simulink model "ijc_template"  (R2020a)
settings: Solver=ode4  StartTime=0.0  StopTime=100  FixedStep=dt  RelTol=1e-3
undefined symbols (not defined in the file): g, Gv, Jm, K, kd1, kd2, ki, kp, Kt, Kv, l1, lc1, lc2, m1, m2, Ra
libraries: simulink x8
settings Model: Creator=baradaran  LastModifiedBy=User
settings DataIOCC: ReturnWorkspaceOutputs=off
settings DebuggingCC: ArithmeticOperatorsInVariantConditions=warning
settings SFSimCC: SimUseLocalCustomCode=off  CustomCodeUndefinedFunction=UseInterfaceOnly
settings RTWCC: RTWUseLocalCustomCode=off

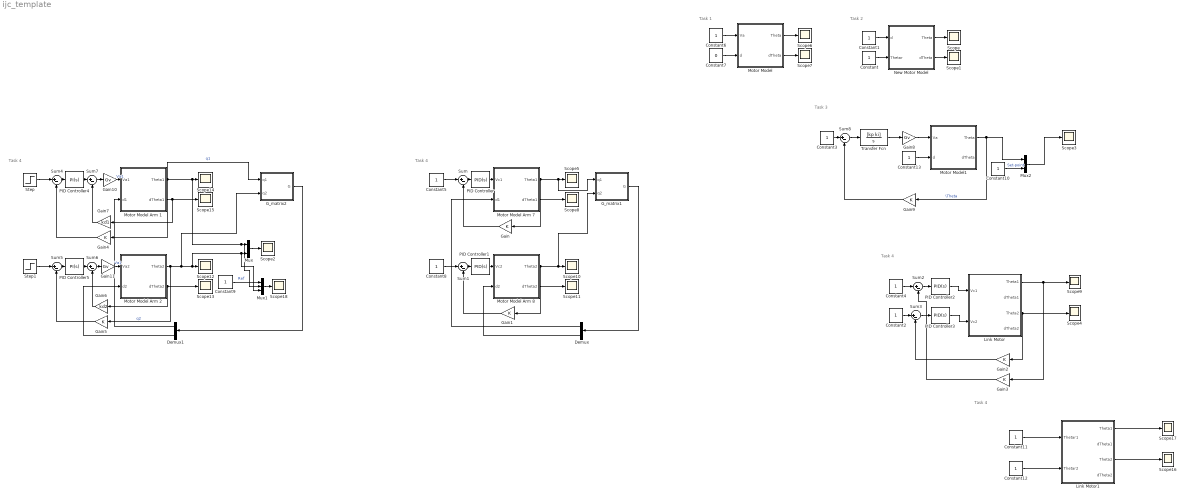
== system ijc_template ==
  note: Task 1
  note: Task 2
  note: Task 3
  note: Task 4
  note: Task 4
  note: Task 4
  note: Task 4
  Constant{,1..6,8..13} (13 alike) : Constant
  Constant7 : Constant  Value=0
  Demux : Demux  Outputs=2
  Demux1 : Demux  Outputs=2
  G_matrix1 : MATLAB Function  TreatAsAtomicUnit=on
  G_matrix2 : MATLAB Function  TreatAsAtomicUnit=on
  Gain{,1..5,9} (7 alike) : Gain  Gain=K
  Gain10 : Gain  Gain=Gv
  Gain11 : Gain  Gain=Gv
  Gain6 : Gain  Gain=kd2
  Gain7 : Gain  Gain=kd1
  Gain8 : Gain  Gain=Gv
  Link Motor : Subsystem
  Link Motor1 : Subsystem
  Motor Model : Subsystem
  Motor Model Arm 1 : Subsystem
  Motor Model Arm 2 : Subsystem
  Motor Model Arm 7 : Subsystem
  Motor Model Arm 8 : Subsystem
  Motor Model1 : Subsystem
  Mux : Mux  Inputs=2
  Mux1 : Mux  Inputs=3
  Mux2 : Mux  Inputs=2
  New Motor Model : Subsystem
  PID Controller : simulink/Continuous/PID Controller  Controller=PID  Form=Parallel  TimeDomain=Continuous-time  UseExternalTs=off  SampleTime=-1  IntegratorMethod=Forward Euler  FilterMethod=Forward Euler  ControllerParametersSource=internal  P=0.930946877105635  I=0.0147921045633956  D=7.75977931127773  UseFilter=on  N=246.215887079108  TunerSelectOption=Transfer Function Based (PID Tuner App)  InitialConditionSource=internal  InitialConditionForIntegrator=0  InitialConditionForFilter=0  DifferentiatorICPrevScaledInput=0  ExternalReset=none  TrackingMode=off  Kt=1  LimitOutput=off  UpperSaturationLimit=inf  LowerSaturationLimit=-inf  LinearizeAsGain=on  AntiWindupMode=none  Kb=1  POutMin=[]  POutMax=[]  IOutMin=[]  IOutMax=[]  DOutMin=[]  DOutMax=[]  NOutMin=[]  NOutMax=[]  SumOutMin=[]  SumOutMax=[]  SaturationOutMin=[]  SaturationOutMax=[]  PParamMin=[]  PParamMax=[]  IParamMin=[]  IParamMax=[]  DParamMin=[]  DParamMax=[]  NParamMin=[]  NParamMax=[]  KbParamMin=[]  KbParamMax=[]  KtParamMin=[]  KtParamMax=[]  KbOutMin=[]  KbOutMax=[]  KtOutMin=[]  KtOutMax=[]  IntegratorOutMin=[]  IntegratorOutMax=[]  FilterOutMin=[]  FilterOutMax=[]  SumI1OutMin=[]  SumI1OutMax=[]  SumI2OutMin=[]  SumI2OutMax=[]  SumI3OutMin=[]  SumI3OutMax=[]  SumI4OutMin=[]  SumI4OutMax=[]  SumDOutMin=[]  SumDOutMax=[]  DifferentiatorOutMin=[]  DifferentiatorOutMax=[]  FilterDiffOutCoefMin=[]  FilterDiffOutCoefMax=[]  ReciprocalOutMin=[]  ReciprocalOutMax=[]  SumDenOutMin=[]  SumDenOutMax=[]  SumNumOutMin=[]  SumNumOutMax=[]  DivideOutMin=[]  DivideOutMax=[]  UdiffTsProdOutMin=[]  UdiffTsProdOutMax=[]  NTsProdOutMin=[]  NTsProdOutMax=[]  UintegralTsProdOutMin=[]  UintegralTsProdOutMax=[]  UngainTsProdOutMin=[]  UngainTsProdOutMax=[]  IntegratorContinuousStateAttributes=''  IntegratorStateMustResolveToSignalObject=off  IntegratorRTWStateStorageClass=Auto  FilterContinuousStateAttributes=''  FilterStateMustResolveToSignalObject=off  FilterRTWStateStorageClass=Auto  ParallelPVariant=InternalParameters  IdealPVariant=Disabled  IVariant=InternalParameters  DVariant=InternalParameters  IntegratorVariant=Continuous  SatVariant=Disabled  AWVariant=Passthrough  PCopyVariant=Disabled  TRVariant=Disabled  FdbkBlocksVariant=Forward  IdealPFdbkVariant=Disabled  SatFdbkVariant=Disabled  DerivativeFilterVariant=ContFilter  NVariant=InternalParameters  NCopyVariant=Disabled  FilterICVariant=InternalICsFilter  IntegratorICVariant=InternalICs  ExternalResetVariant=Disabled  TRSumVariant=Passthrough  SumFdbkVariant=Disabled  SumVariant=Sum_PID  TsampFilterVariant=InternalTs  TsampNgainVariant=Passthrough  TsampIntegralVariant=Passthrough
  PID Controller1 : simulink/Continuous/PID Controller  Controller=PID  Form=Parallel  TimeDomain=Continuous-time  UseExternalTs=off  SampleTime=-1  IntegratorMethod=Forward Euler  FilterMethod=Forward Euler  ControllerParametersSource=internal  P=2.05230047668666  I=0.193213957574271  D=4.85797869195196  UseFilter=on  N=7.76332869091656  TunerSelectOption=Transfer Function Based (PID Tuner App)  InitialConditionSource=internal  InitialConditionForIntegrator=0  InitialConditionForFilter=0  DifferentiatorICPrevScaledInput=0  ExternalReset=none  TrackingMode=off  Kt=1  LimitOutput=off  UpperSaturationLimit=inf  LowerSaturationLimit=-inf  LinearizeAsGain=on  AntiWindupMode=none  Kb=1  POutMin=[]  POutMax=[]  IOutMin=[]  IOutMax=[]  DOutMin=[]  DOutMax=[]  NOutMin=[]  NOutMax=[]  SumOutMin=[]  SumOutMax=[]  SaturationOutMin=[]  SaturationOutMax=[]  PParamMin=[]  PParamMax=[]  IParamMin=[]  IParamMax=[]  DParamMin=[]  DParamMax=[]  NParamMin=[]  NParamMax=[]  KbParamMin=[]  KbParamMax=[]  KtParamMin=[]  KtParamMax=[]  KbOutMin=[]  KbOutMax=[]  KtOutMin=[]  KtOutMax=[]  IntegratorOutMin=[]  IntegratorOutMax=[]  FilterOutMin=[]  FilterOutMax=[]  SumI1OutMin=[]  SumI1OutMax=[]  SumI2OutMin=[]  SumI2OutMax=[]  SumI3OutMin=[]  SumI3OutMax=[]  SumI4OutMin=[]  SumI4OutMax=[]  SumDOutMin=[]  SumDOutMax=[]  DifferentiatorOutMin=[]  DifferentiatorOutMax=[]  FilterDiffOutCoefMin=[]  FilterDiffOutCoefMax=[]  ReciprocalOutMin=[]  ReciprocalOutMax=[]  SumDenOutMin=[]  SumDenOutMax=[]  SumNumOutMin=[]  SumNumOutMax=[]  DivideOutMin=[]  DivideOutMax=[]  UdiffTsProdOutMin=[]  UdiffTsProdOutMax=[]  NTsProdOutMin=[]  NTsProdOutMax=[]  UintegralTsProdOutMin=[]  UintegralTsProdOutMax=[]  UngainTsProdOutMin=[]  UngainTsProdOutMax=[]  IntegratorContinuousStateAttributes=''  IntegratorStateMustResolveToSignalObject=off  IntegratorRTWStateStorageClass=Auto  FilterContinuousStateAttributes=''  FilterStateMustResolveToSignalObject=off  FilterRTWStateStorageClass=Auto  ParallelPVariant=InternalParameters  IdealPVariant=Disabled  IVariant=InternalParameters  DVariant=InternalParameters  IntegratorVariant=Continuous  SatVariant=Disabled  AWVariant=Passthrough  PCopyVariant=Disabled  TRVariant=Disabled  FdbkBlocksVariant=Forward  IdealPFdbkVariant=Disabled  SatFdbkVariant=Disabled  DerivativeFilterVariant=ContFilter  NVariant=InternalParameters  NCopyVariant=Disabled  FilterICVariant=InternalICsFilter  IntegratorICVariant=InternalICs  ExternalResetVariant=Disabled  TRSumVariant=Passthrough  SumFdbkVariant=Disabled  SumVariant=Sum_PID  TsampFilterVariant=InternalTs  TsampNgainVariant=Passthrough  TsampIntegralVariant=Passthrough
  PID Controller2 : simulink/Continuous/PID Controller  Controller=PID  Form=Parallel  TimeDomain=Continuous-time  UseExternalTs=off  SampleTime=-1  IntegratorMethod=Forward Euler  FilterMethod=Forward Euler  ControllerParametersSource=internal  P=1.76218058045998  I=0.160161970313347  D=4.42256720498161  UseFilter=on  N=7.08023991559863  TunerSelectOption=Transfer Function Based (PID Tuner App)  InitialConditionSource=internal  InitialConditionForIntegrator=0  InitialConditionForFilter=0  DifferentiatorICPrevScaledInput=0  ExternalReset=none  TrackingMode=off  Kt=1  LimitOutput=off  UpperSaturationLimit=inf  LowerSaturationLimit=-inf  LinearizeAsGain=on  AntiWindupMode=none  Kb=1  POutMin=[]  POutMax=[]  IOutMin=[]  IOutMax=[]  DOutMin=[]  DOutMax=[]  NOutMin=[]  NOutMax=[]  SumOutMin=[]  SumOutMax=[]  SaturationOutMin=[]  SaturationOutMax=[]  PParamMin=[]  PParamMax=[]  IParamMin=[]  IParamMax=[]  DParamMin=[]  DParamMax=[]  NParamMin=[]  NParamMax=[]  KbParamMin=[]  KbParamMax=[]  KtParamMin=[]  KtParamMax=[]  KbOutMin=[]  KbOutMax=[]  KtOutMin=[]  KtOutMax=[]  IntegratorOutMin=[]  IntegratorOutMax=[]  FilterOutMin=[]  FilterOutMax=[]  SumI1OutMin=[]  SumI1OutMax=[]  SumI2OutMin=[]  SumI2OutMax=[]  SumI3OutMin=[]  SumI3OutMax=[]  SumI4OutMin=[]  SumI4OutMax=[]  SumDOutMin=[]  SumDOutMax=[]  DifferentiatorOutMin=[]  DifferentiatorOutMax=[]  FilterDiffOutCoefMin=[]  FilterDiffOutCoefMax=[]  ReciprocalOutMin=[]  ReciprocalOutMax=[]  SumDenOutMin=[]  SumDenOutMax=[]  SumNumOutMin=[]  SumNumOutMax=[]  DivideOutMin=[]  DivideOutMax=[]  UdiffTsProdOutMin=[]  UdiffTsProdOutMax=[]  NTsProdOutMin=[]  NTsProdOutMax=[]  UintegralTsProdOutMin=[]  UintegralTsProdOutMax=[]  UngainTsProdOutMin=[]  UngainTsProdOutMax=[]  IntegratorContinuousStateAttributes=''  IntegratorStateMustResolveToSignalObject=off  IntegratorRTWStateStorageClass=Auto  FilterContinuousStateAttributes=''  FilterStateMustResolveToSignalObject=off  FilterRTWStateStorageClass=Auto  ParallelPVariant=InternalParameters  IdealPVariant=Disabled  IVariant=InternalParameters  DVariant=InternalParameters  IntegratorVariant=Continuous  SatVariant=Disabled  AWVariant=Passthrough  PCopyVariant=Disabled  TRVariant=Disabled  FdbkBlocksVariant=Forward  IdealPFdbkVariant=Disabled  SatFdbkVariant=Disabled  DerivativeFilterVariant=ContFilter  NVariant=InternalParameters  NCopyVariant=Disabled  FilterICVariant=InternalICsFilter  IntegratorICVariant=InternalICs  ExternalResetVariant=Disabled  TRSumVariant=Passthrough  SumFdbkVariant=Disabled  SumVariant=Sum_PID  TsampFilterVariant=InternalTs  TsampNgainVariant=Passthrough  TsampIntegralVariant=Passthrough
  PID Controller3 : simulink/Continuous/PID Controller  Controller=PID  Form=Parallel  TimeDomain=Continuous-time  UseExternalTs=off  SampleTime=-1  IntegratorMethod=Forward Euler  FilterMethod=Forward Euler  ControllerParametersSource=internal  P=2.15820002385738  I=0.146873136290842  D=4.7214823808971  UseFilter=on  N=155.351722280269  TunerSelectOption=Transfer Function Based (PID Tuner App)  InitialConditionSource=internal  InitialConditionForIntegrator=0  InitialConditionForFilter=0  DifferentiatorICPrevScaledInput=0  ExternalReset=none  TrackingMode=off  Kt=1  LimitOutput=off  UpperSaturationLimit=inf  LowerSaturationLimit=-inf  LinearizeAsGain=on  AntiWindupMode=none  Kb=1  POutMin=[]  POutMax=[]  IOutMin=[]  IOutMax=[]  DOutMin=[]  DOutMax=[]  NOutMin=[]  NOutMax=[]  SumOutMin=[]  SumOutMax=[]  SaturationOutMin=[]  SaturationOutMax=[]  PParamMin=[]  PParamMax=[]  IParamMin=[]  IParamMax=[]  DParamMin=[]  DParamMax=[]  NParamMin=[]  NParamMax=[]  KbParamMin=[]  KbParamMax=[]  KtParamMin=[]  KtParamMax=[]  KbOutMin=[]  KbOutMax=[]  KtOutMin=[]  KtOutMax=[]  IntegratorOutMin=[]  IntegratorOutMax=[]  FilterOutMin=[]  FilterOutMax=[]  SumI1OutMin=[]  SumI1OutMax=[]  SumI2OutMin=[]  SumI2OutMax=[]  SumI3OutMin=[]  SumI3OutMax=[]  SumI4OutMin=[]  SumI4OutMax=[]  SumDOutMin=[]  SumDOutMax=[]  DifferentiatorOutMin=[]  DifferentiatorOutMax=[]  FilterDiffOutCoefMin=[]  FilterDiffOutCoefMax=[]  ReciprocalOutMin=[]  ReciprocalOutMax=[]  SumDenOutMin=[]  SumDenOutMax=[]  SumNumOutMin=[]  SumNumOutMax=[]  DivideOutMin=[]  DivideOutMax=[]  UdiffTsProdOutMin=[]  UdiffTsProdOutMax=[]  NTsProdOutMin=[]  NTsProdOutMax=[]  UintegralTsProdOutMin=[]  UintegralTsProdOutMax=[]  UngainTsProdOutMin=[]  UngainTsProdOutMax=[]  IntegratorContinuousStateAttributes=''  IntegratorStateMustResolveToSignalObject=off  IntegratorRTWStateStorageClass=Auto  FilterContinuousStateAttributes=''  FilterStateMustResolveToSignalObject=off  FilterRTWStateStorageClass=Auto  ParallelPVariant=InternalParameters  IdealPVariant=Disabled  IVariant=InternalParameters  DVariant=InternalParameters  IntegratorVariant=Continuous  SatVariant=Disabled  AWVariant=Passthrough  PCopyVariant=Disabled  TRVariant=Disabled  FdbkBlocksVariant=Forward  IdealPFdbkVariant=Disabled  SatFdbkVariant=Disabled  DerivativeFilterVariant=ContFilter  NVariant=InternalParameters  NCopyVariant=Disabled  FilterICVariant=InternalICsFilter  IntegratorICVariant=InternalICs  ExternalResetVariant=Disabled  TRSumVariant=Passthrough  SumFdbkVariant=Disabled  SumVariant=Sum_PID  TsampFilterVariant=InternalTs  TsampNgainVariant=Passthrough  TsampIntegralVariant=Passthrough
  PID Controller4 : simulink/Continuous/PID Controller  Controller=PI  Form=Parallel  TimeDomain=Continuous-time  UseExternalTs=off  SampleTime=-1  IntegratorMethod=Forward Euler  FilterMethod=Forward Euler  ControllerParametersSource=internal  P=696.299096239022  I=132.737691368979  D=13.9952614097223  UseFilter=on  N=461.197118668005  TunerSelectOption=Transfer Function Based (PID Tuner App)  InitialConditionSource=internal  InitialConditionForIntegrator=0  InitialConditionForFilter=0  DifferentiatorICPrevScaledInput=0  ExternalReset=none  TrackingMode=off  Kt=1  LimitOutput=off  UpperSaturationLimit=inf  LowerSaturationLimit=-inf  LinearizeAsGain=on  AntiWindupMode=none  Kb=1  POutMin=[]  POutMax=[]  IOutMin=[]  IOutMax=[]  DOutMin=[]  DOutMax=[]  NOutMin=[]  NOutMax=[]  SumOutMin=[]  SumOutMax=[]  SaturationOutMin=[]  SaturationOutMax=[]  PParamMin=[]  PParamMax=[]  IParamMin=[]  IParamMax=[]  DParamMin=[]  DParamMax=[]  NParamMin=[]  NParamMax=[]  KbParamMin=[]  KbParamMax=[]  KtParamMin=[]  KtParamMax=[]  KbOutMin=[]  KbOutMax=[]  KtOutMin=[]  KtOutMax=[]  IntegratorOutMin=[]  IntegratorOutMax=[]  FilterOutMin=[]  FilterOutMax=[]  SumI1OutMin=[]  SumI1OutMax=[]  SumI2OutMin=[]  SumI2OutMax=[]  SumI3OutMin=[]  SumI3OutMax=[]  SumI4OutMin=[]  SumI4OutMax=[]  SumDOutMin=[]  SumDOutMax=[]  DifferentiatorOutMin=[]  DifferentiatorOutMax=[]  FilterDiffOutCoefMin=[]  FilterDiffOutCoefMax=[]  ReciprocalOutMin=[]  ReciprocalOutMax=[]  SumDenOutMin=[]  SumDenOutMax=[]  SumNumOutMin=[]  SumNumOutMax=[]  DivideOutMin=[]  DivideOutMax=[]  UdiffTsProdOutMin=[]  UdiffTsProdOutMax=[]  NTsProdOutMin=[]  NTsProdOutMax=[]  UintegralTsProdOutMin=[]  UintegralTsProdOutMax=[]  UngainTsProdOutMin=[]  UngainTsProdOutMax=[]  IntegratorContinuousStateAttributes=''  IntegratorStateMustResolveToSignalObject=off  IntegratorRTWStateStorageClass=Auto  FilterContinuousStateAttributes=''  FilterStateMustResolveToSignalObject=off  FilterRTWStateStorageClass=Auto  ParallelPVariant=InternalParameters  IdealPVariant=Disabled  IVariant=InternalParameters  DVariant=Disabled  IntegratorVariant=Continuous  SatVariant=Disabled  AWVariant=Passthrough  PCopyVariant=Disabled  TRVariant=Disabled  FdbkBlocksVariant=Forward  IdealPFdbkVariant=Disabled  SatFdbkVariant=Disabled  DerivativeFilterVariant=Disabled  NVariant=Disabled  NCopyVariant=Disabled_SignalSpec  FilterICVariant=Disabled  IntegratorICVariant=InternalICs  ExternalResetVariant=Disabled  TRSumVariant=Passthrough  SumFdbkVariant=Disabled  SumVariant=Sum_PI  TsampFilterVariant=InternalTs  TsampNgainVariant=Passthrough  TsampIntegralVariant=Passthrough
  PID Controller5 : simulink/Continuous/PID Controller  Controller=PI  Form=Parallel  TimeDomain=Continuous-time  UseExternalTs=off  SampleTime=-1  IntegratorMethod=Forward Euler  FilterMethod=Forward Euler  ControllerParametersSource=internal  P=74.5518923678732  I=31.5791033290128  D=5.86455505756343  UseFilter=on  N=9.33357397933394  TunerSelectOption=Transfer Function Based (PID Tuner App)  InitialConditionSource=internal  InitialConditionForIntegrator=0  InitialConditionForFilter=0  DifferentiatorICPrevScaledInput=0  ExternalReset=none  TrackingMode=off  Kt=1  LimitOutput=off  UpperSaturationLimit=inf  LowerSaturationLimit=-inf  LinearizeAsGain=on  AntiWindupMode=none  Kb=1  POutMin=[]  POutMax=[]  IOutMin=[]  IOutMax=[]  DOutMin=[]  DOutMax=[]  NOutMin=[]  NOutMax=[]  SumOutMin=[]  SumOutMax=[]  SaturationOutMin=[]  SaturationOutMax=[]  PParamMin=[]  PParamMax=[]  IParamMin=[]  IParamMax=[]  DParamMin=[]  DParamMax=[]  NParamMin=[]  NParamMax=[]  KbParamMin=[]  KbParamMax=[]  KtParamMin=[]  KtParamMax=[]  KbOutMin=[]  KbOutMax=[]  KtOutMin=[]  KtOutMax=[]  IntegratorOutMin=[]  IntegratorOutMax=[]  FilterOutMin=[]  FilterOutMax=[]  SumI1OutMin=[]  SumI1OutMax=[]  SumI2OutMin=[]  SumI2OutMax=[]  SumI3OutMin=[]  SumI3OutMax=[]  SumI4OutMin=[]  SumI4OutMax=[]  SumDOutMin=[]  SumDOutMax=[]  DifferentiatorOutMin=[]  DifferentiatorOutMax=[]  FilterDiffOutCoefMin=[]  FilterDiffOutCoefMax=[]  ReciprocalOutMin=[]  ReciprocalOutMax=[]  SumDenOutMin=[]  SumDenOutMax=[]  SumNumOutMin=[]  SumNumOutMax=[]  DivideOutMin=[]  DivideOutMax=[]  UdiffTsProdOutMin=[]  UdiffTsProdOutMax=[]  NTsProdOutMin=[]  NTsProdOutMax=[]  UintegralTsProdOutMin=[]  UintegralTsProdOutMax=[]  UngainTsProdOutMin=[]  UngainTsProdOutMax=[]  IntegratorContinuousStateAttributes=''  IntegratorStateMustResolveToSignalObject=off  IntegratorRTWStateStorageClass=Auto  FilterContinuousStateAttributes=''  FilterStateMustResolveToSignalObject=off  FilterRTWStateStorageClass=Auto  ParallelPVariant=InternalParameters  IdealPVariant=Disabled  IVariant=InternalParameters  DVariant=Disabled  IntegratorVariant=Continuous  SatVariant=Disabled  AWVariant=Passthrough  PCopyVariant=Disabled  TRVariant=Disabled  FdbkBlocksVariant=Forward  IdealPFdbkVariant=Disabled  SatFdbkVariant=Disabled  DerivativeFilterVariant=Disabled  NVariant=Disabled  NCopyVariant=Disabled_SignalSpec  FilterICVariant=Disabled  IntegratorICVariant=InternalICs  ExternalResetVariant=Disabled  TRSumVariant=Passthrough  SumFdbkVariant=Disabled  SumVariant=Sum_PI  TsampFilterVariant=InternalTs  TsampNgainVariant=Passthrough  TsampIntegralVariant=Passthrough
  Scope{,1..18} (19 alike) : Scope
  Step : Step  SampleTime=0
  Step1 : Step  SampleTime=0
  Sum{,1..8} (9 alike) : Sum  Inputs=|+-
  Transfer Fcn : TransferFcn  Numerator=[kp ki]  Denominator=[1 0]
  wires:
  Constant6/1 -> Motor Model/1(Va)
  Constant7/1 -> Motor Model/2(d)
  Motor Model/1(Theta) -> Scope6/1
  Motor Model/2(dTheta) -> Scope7/1
  New Motor Model/1(Theta) -> Scope/1
  New Motor Model/2(dTheta) -> Scope1/1
  Constant/1 -> New Motor Model/2(Thetar)
  Constant1/1 -> New Motor Model/1(d)
  Link Motor/1(Theta1) -> Gain3/1, Scope9/1
  Link Motor/3(Theta2) -> Gain2/1, Scope4/1
  Motor Model Arm 7/1(Theta1) -> Gain/1, G_matrix1/1(q1), Scope5/1
  Motor Model Arm 7/2(dTheta1) -> Scope8/1
  Sum/1 -> PID Controller/1
  PID Controller/1 -> Motor Model Arm 7/1(Vc1)
  Constant5/1 -> Sum/1
  Motor Model Arm 8/2(dTheta2) -> Scope11/1
  Constant8/1 -> Sum1/1
  Sum1/1 -> PID Controller1/1
  Motor Model Arm 8/1(Theta2) -> Gain1/1, G_matrix1/2(q2), Scope10/1
  G_matrix1/1(G) -> Demux/1
  Demux/1 -> Motor Model Arm 7/2(d1)
  Demux/2 -> Motor Model Arm 8/2(d2)
  Gain/1 -> Sum/2
  Gain1/1 -> Sum1/2
  PID Controller1/1 -> Motor Model Arm 8/1(Vc2)
  PID Controller2/1 -> Link Motor/1(Vc1)
  PID Controller3/1 -> Link Motor/2(Vc2)
  Constant4/1 -> Sum2/1
  Sum2/1 -> PID Controller2/1
  Constant2/1 -> Sum3/1
  Sum3/1 -> PID Controller3/1
  Gain2/1 -> Sum3/2
  Gain3/1 -> Sum2/2
  Step1/1 -> Sum5/1
  Step/1 -> Sum4/1
  Demux1/2 -> Motor Model Arm 2/2(d2)
  Sum5/1 -> PID Controller5/1
  Sum4/1 -> PID Controller4/1
  Gain5/1 -> Sum5/2
  Gain4/1 -> Sum4/2
  G_matrix2/1(G) -> Demux1/1
  Motor Model Arm 1/1(Theta1) -> Gain4/1, G_matrix2/1(q1), Mux1/2, Mux/1, Scope14/1  "q1"
  Motor Model Arm 1/2(dTheta1) -> Gain7/1, Scope15/1
  Motor Model Arm 2/1(Theta2) -> G_matrix2/2(q2), Mux1/3, Mux/2, Scope12/1, Gain5/1  "q2"
  Motor Model Arm 2/2(dTheta2) -> Gain6/1, Scope13/1
  PID Controller4/1 -> Sum7/1
  Link Motor1/3(Theta2) -> Scope16/1
  Link Motor1/1(Theta1) -> Scope17/1
  Constant11/1 -> Link Motor1/1(Thetar1)
  Constant12/1 -> Link Motor1/2(Thetar2)
  PID Controller5/1 -> Sum6/1
  Gain6/1 -> Sum6/2
  Gain7/1 -> Sum7/2
  Demux1/1 -> Motor Model Arm 1/2(d1)
  Mux/1 -> Scope2/1
  Gain8/1 -> Motor Model1/1(Va)
  Transfer Fcn/1 -> Gain8/1
  Motor Model1/1(Theta) -> Mux2/1, Gain9/1  "\\Theta"
  Sum8/1 -> Transfer Fcn/1
  Gain9/1 -> Sum8/2
  Constant3/1 -> Sum8/1
  Constant13/1 -> Motor Model1/2(d)
  Sum7/1 -> Gain10/1
  Gain10/1 -> Motor Model Arm 1/1(Va1)  "Va1"
  Sum6/1 -> Gain11/1
  Gain11/1 -> Motor Model Arm 2/1(Va2)  "Va1"
  Constant9/1 -> Mux1/1  "Ref"
  Mux1/1 -> Scope18/1
  Constant10/1 -> Mux2/2  "Set-point"
  Mux2/1 -> Scope3/1

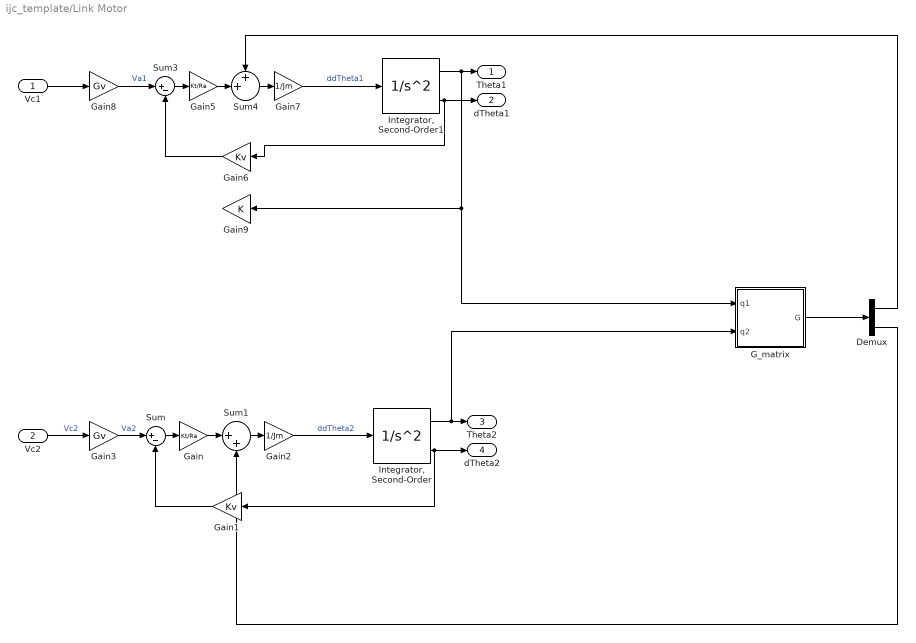
== system ijc_template/Link Motor ==
  Vc1 : Inport
  Vc2 : Inport  Port=2
  Demux : Demux  Outputs=2
  G_matrix : MATLAB Function  TreatAsAtomicUnit=on
  Gain : Gain  Gain=Kt/Ra
  Gain1 : Gain  Gain=Kv
  Gain2 : Gain  Gain=1/Jm
  Gain3 : Gain  Gain=Gv
  Gain5 : Gain  Gain=Kt/Ra
  Gain6 : Gain  Gain=Kv
  Gain7 : Gain  Gain=1/Jm
  Gain8 : Gain  Gain=Gv
  Gain9 : Gain  Gain=K
  "Integrator, Second-Order" : SecondOrderIntegrator
  "Integrator, Second-Order1" : SecondOrderIntegrator
  Sum : Sum  Inputs=|+-
  Sum1 : Sum  Inputs=|++
  Sum3 : Sum  Inputs=|+-
  Sum4 : Sum  Inputs=++|
  Theta1 : Outport
  dTheta1 : Outport  Port=2
  Theta2 : Outport  Port=3
  dTheta2 : Outport  Port=4
  wires:
  Sum/1 -> Gain/1
  "Integrator, Second-Order"/1 -> Theta2/1, G_matrix/2(q2)
  "Integrator, Second-Order"/2 -> dTheta2/1, Gain1/1
  Gain1/1 -> Sum/2
  Gain3/1 -> Sum/1  "Va2"
  Gain/1 -> Sum1/1
  Sum1/1 -> Gain2/1
  Gain2/1 -> "Integrator, Second-Order"/1  "ddTheta2"
  Sum4/1 -> Gain7/1
  Gain6/1 -> Sum3/2
  Gain8/1 -> Sum3/1  "Va1"
  Gain7/1 -> "Integrator, Second-Order1"/1  "ddTheta1"
  Sum3/1 -> Gain5/1
  "Integrator, Second-Order1"/1 -> Gain9/1, G_matrix/1(q1), Theta1/1
  "Integrator, Second-Order1"/2 -> dTheta1/1, Gain6/1
  Vc2/1 -> Gain3/1  "Vc2"
  Gain5/1 -> Sum4/2
  Demux/1 -> Sum4/1
  Demux/2 -> Sum1/2
  G_matrix/1(G) -> Demux/1
  Vc1/1 -> Gain8/1

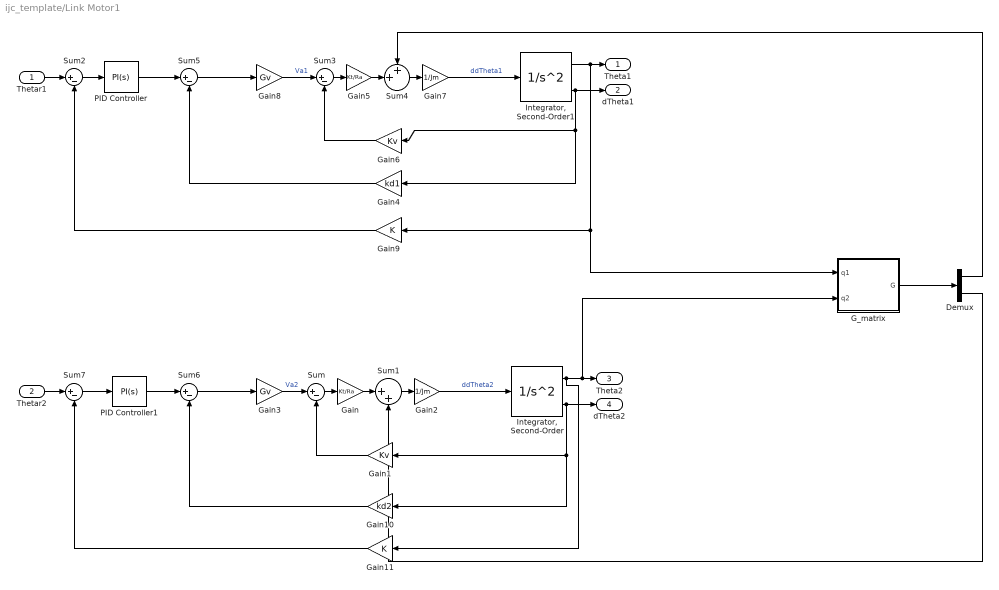
== system ijc_template/Link Motor1 ==
  Thetar1 : Inport
  Thetar2 : Inport  Port=2
  Demux : Demux  Outputs=2
  G_matrix : MATLAB Function  TreatAsAtomicUnit=on
  Gain : Gain  Gain=Kt/Ra
  Gain1 : Gain  Gain=Kv
  Gain10 : Gain  Gain=kd2
  Gain11 : Gain  Gain=K
  Gain2 : Gain  Gain=1/Jm
  Gain3 : Gain  Gain=Gv
  Gain4 : Gain  Gain=kd1
  Gain5 : Gain  Gain=Kt/Ra
  Gain6 : Gain  Gain=Kv
  Gain7 : Gain  Gain=1/Jm
  Gain8 : Gain  Gain=Gv
  Gain9 : Gain  Gain=K
  "Integrator, Second-Order" : SecondOrderIntegrator
  "Integrator, Second-Order1" : SecondOrderIntegrator
  PID Controller : simulink/Continuous/PID Controller  Controller=PI  Form=Parallel  TimeDomain=Continuous-time  UseExternalTs=off  SampleTime=-1  IntegratorMethod=Forward Euler  FilterMethod=Forward Euler  ControllerParametersSource=internal  P=1.70873528824987  I=0.0146792238569882  D=0  UseFilter=on  N=100  TunerSelectOption=Transfer Function Based (PID Tuner App)  InitialConditionSource=internal  InitialConditionForIntegrator=0  InitialConditionForFilter=0  DifferentiatorICPrevScaledInput=0  ExternalReset=none  TrackingMode=off  Kt=1  LimitOutput=off  UpperSaturationLimit=inf  LowerSaturationLimit=-inf  LinearizeAsGain=on  AntiWindupMode=none  Kb=1  POutMin=[]  POutMax=[]  IOutMin=[]  IOutMax=[]  DOutMin=[]  DOutMax=[]  NOutMin=[]  NOutMax=[]  SumOutMin=[]  SumOutMax=[]  SaturationOutMin=[]  SaturationOutMax=[]  PParamMin=[]  PParamMax=[]  IParamMin=[]  IParamMax=[]  DParamMin=[]  DParamMax=[]  NParamMin=[]  NParamMax=[]  KbParamMin=[]  KbParamMax=[]  KtParamMin=[]  KtParamMax=[]  KbOutMin=[]  KbOutMax=[]  KtOutMin=[]  KtOutMax=[]  IntegratorOutMin=[]  IntegratorOutMax=[]  FilterOutMin=[]  FilterOutMax=[]  SumI1OutMin=[]  SumI1OutMax=[]  SumI2OutMin=[]  SumI2OutMax=[]  SumI3OutMin=[]  SumI3OutMax=[]  SumI4OutMin=[]  SumI4OutMax=[]  SumDOutMin=[]  SumDOutMax=[]  DifferentiatorOutMin=[]  DifferentiatorOutMax=[]  FilterDiffOutCoefMin=[]  FilterDiffOutCoefMax=[]  ReciprocalOutMin=[]  ReciprocalOutMax=[]  SumDenOutMin=[]  SumDenOutMax=[]  SumNumOutMin=[]  SumNumOutMax=[]  DivideOutMin=[]  DivideOutMax=[]  UdiffTsProdOutMin=[]  UdiffTsProdOutMax=[]  NTsProdOutMin=[]  NTsProdOutMax=[]  UintegralTsProdOutMin=[]  UintegralTsProdOutMax=[]  UngainTsProdOutMin=[]  UngainTsProdOutMax=[]  IntegratorContinuousStateAttributes=''  IntegratorStateMustResolveToSignalObject=off  IntegratorRTWStateStorageClass=Auto  FilterContinuousStateAttributes=''  FilterStateMustResolveToSignalObject=off  FilterRTWStateStorageClass=Auto  ParallelPVariant=InternalParameters  IdealPVariant=Disabled  IVariant=InternalParameters  DVariant=Disabled  IntegratorVariant=Continuous  SatVariant=Disabled  AWVariant=Passthrough  PCopyVariant=Disabled  TRVariant=Disabled  FdbkBlocksVariant=Forward  IdealPFdbkVariant=Disabled  SatFdbkVariant=Disabled  DerivativeFilterVariant=Disabled  NVariant=Disabled  NCopyVariant=Disabled_SignalSpec  FilterICVariant=Disabled  IntegratorICVariant=InternalICs  ExternalResetVariant=Disabled  TRSumVariant=Passthrough  SumFdbkVariant=Disabled  SumVariant=Sum_PI  TsampFilterVariant=InternalTs  TsampNgainVariant=Passthrough  TsampIntegralVariant=Passthrough
  PID Controller1 : simulink/Continuous/PID Controller  Controller=PI  Form=Parallel  TimeDomain=Continuous-time  UseExternalTs=off  SampleTime=-1  IntegratorMethod=Forward Euler  FilterMethod=Forward Euler  ControllerParametersSource=internal  P=1.92177703343693  I=0.0181021977148352  D=0  UseFilter=on  N=100  TunerSelectOption=Transfer Function Based (PID Tuner App)  InitialConditionSource=internal  InitialConditionForIntegrator=0  InitialConditionForFilter=0  DifferentiatorICPrevScaledInput=0  ExternalReset=none  TrackingMode=off  Kt=1  LimitOutput=off  UpperSaturationLimit=inf  LowerSaturationLimit=-inf  LinearizeAsGain=on  AntiWindupMode=none  Kb=1  POutMin=[]  POutMax=[]  IOutMin=[]  IOutMax=[]  DOutMin=[]  DOutMax=[]  NOutMin=[]  NOutMax=[]  SumOutMin=[]  SumOutMax=[]  SaturationOutMin=[]  SaturationOutMax=[]  PParamMin=[]  PParamMax=[]  IParamMin=[]  IParamMax=[]  DParamMin=[]  DParamMax=[]  NParamMin=[]  NParamMax=[]  KbParamMin=[]  KbParamMax=[]  KtParamMin=[]  KtParamMax=[]  KbOutMin=[]  KbOutMax=[]  KtOutMin=[]  KtOutMax=[]  IntegratorOutMin=[]  IntegratorOutMax=[]  FilterOutMin=[]  FilterOutMax=[]  SumI1OutMin=[]  SumI1OutMax=[]  SumI2OutMin=[]  SumI2OutMax=[]  SumI3OutMin=[]  SumI3OutMax=[]  SumI4OutMin=[]  SumI4OutMax=[]  SumDOutMin=[]  SumDOutMax=[]  DifferentiatorOutMin=[]  DifferentiatorOutMax=[]  FilterDiffOutCoefMin=[]  FilterDiffOutCoefMax=[]  ReciprocalOutMin=[]  ReciprocalOutMax=[]  SumDenOutMin=[]  SumDenOutMax=[]  SumNumOutMin=[]  SumNumOutMax=[]  DivideOutMin=[]  DivideOutMax=[]  UdiffTsProdOutMin=[]  UdiffTsProdOutMax=[]  NTsProdOutMin=[]  NTsProdOutMax=[]  UintegralTsProdOutMin=[]  UintegralTsProdOutMax=[]  UngainTsProdOutMin=[]  UngainTsProdOutMax=[]  IntegratorContinuousStateAttributes=''  IntegratorStateMustResolveToSignalObject=off  IntegratorRTWStateStorageClass=Auto  FilterContinuousStateAttributes=''  FilterStateMustResolveToSignalObject=off  FilterRTWStateStorageClass=Auto  ParallelPVariant=InternalParameters  IdealPVariant=Disabled  IVariant=InternalParameters  DVariant=Disabled  IntegratorVariant=Continuous  SatVariant=Disabled  AWVariant=Passthrough  PCopyVariant=Disabled  TRVariant=Disabled  FdbkBlocksVariant=Forward  IdealPFdbkVariant=Disabled  SatFdbkVariant=Disabled  DerivativeFilterVariant=Disabled  NVariant=Disabled  NCopyVariant=Disabled_SignalSpec  FilterICVariant=Disabled  IntegratorICVariant=InternalICs  ExternalResetVariant=Disabled  TRSumVariant=Passthrough  SumFdbkVariant=Disabled  SumVariant=Sum_PI  TsampFilterVariant=InternalTs  TsampNgainVariant=Passthrough  TsampIntegralVariant=Passthrough
  Sum{,2..3,5..7} (6 alike) : Sum  Inputs=|+-
  Sum1 : Sum  Inputs=|++
  Sum4 : Sum  Inputs=++|
  Theta1 : Outport
  dTheta1 : Outport  Port=2
  Theta2 : Outport  Port=3
  dTheta2 : Outport  Port=4
  wires:
  Sum/1 -> Gain/1
  "Integrator, Second-Order"/1 -> Gain11/1, Theta2/1, G_matrix/2(q2)
  "Integrator, Second-Order"/2 -> dTheta2/1, Gain1/1, Gain10/1
  Gain1/1 -> Sum/2
  Gain3/1 -> Sum/1  "Va2"
  Gain/1 -> Sum1/1
  Sum1/1 -> Gain2/1
  Gain2/1 -> "Integrator, Second-Order"/1  "ddTheta2"
  Sum4/1 -> Gain7/1
  Gain6/1 -> Sum3/2
  Gain8/1 -> Sum3/1  "Va1"
  Gain7/1 -> "Integrator, Second-Order1"/1  "ddTheta1"
  Sum3/1 -> Gain5/1
  "Integrator, Second-Order1"/1 -> Gain9/1, G_matrix/1(q1), Theta1/1
  "Integrator, Second-Order1"/2 -> Gain6/1, Gain4/1, dTheta1/1
  Gain5/1 -> Sum4/2
  Demux/1 -> Sum4/1
  Demux/2 -> Sum1/2
  G_matrix/1(G) -> Demux/1
  Thetar1/1 -> Sum2/1
  Sum2/1 -> PID Controller/1
  Gain9/1 -> Sum2/2
  Gain4/1 -> Sum5/2
  PID Controller/1 -> Sum5/1
  Sum5/1 -> Gain8/1
  Thetar2/1 -> Sum7/1
  Gain10/1 -> Sum6/2
  Sum7/1 -> PID Controller1/1
  PID Controller1/1 -> Sum6/1
  Sum6/1 -> Gain3/1
  Gain11/1 -> Sum7/2

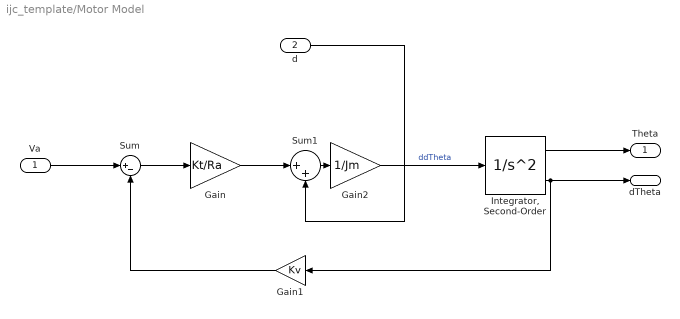
== system ijc_template/Motor Model ==
  Va : Inport
  d : Inport  Port=2
  Gain : Gain  Gain=Kt/Ra
  Gain1 : Gain  Gain=Kv
  Gain2 : Gain  Gain=1/Jm
  "Integrator, Second-Order" : SecondOrderIntegrator
  Sum : Sum  Inputs=|+-
  Sum1 : Sum  Inputs=|++
  Theta : Outport  VectorParamsAs1DForOutWhenUnconnected=off
  dTheta : Outport  Port=2  VectorParamsAs1DForOutWhenUnconnected=off
  wires:
  Sum/1 -> Gain/1
  "Integrator, Second-Order"/1 -> Theta/1
  d/1 -> Sum1/2
  Gain1/1 -> Sum/2
  Va/1 -> Sum/1
  Gain/1 -> Sum1/1
  Sum1/1 -> Gain2/1
  Gain2/1 -> "Integrator, Second-Order"/1  "ddTheta"
  "Integrator, Second-Order"/2 -> Gain1/1, dTheta/1

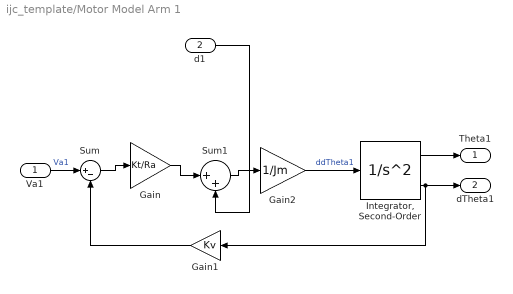
== system ijc_template/Motor Model Arm 1 ==
  Va1 : Inport
  d1 : Inport  Port=2
  Gain : Gain  Gain=Kt/Ra
  Gain1 : Gain  Gain=Kv
  Gain2 : Gain  Gain=1/Jm
  "Integrator, Second-Order" : SecondOrderIntegrator
  Sum : Sum  Inputs=|+-
  Sum1 : Sum  Inputs=|++
  Theta1 : Outport  VectorParamsAs1DForOutWhenUnconnected=off
  dTheta1 : Outport  Port=2  VectorParamsAs1DForOutWhenUnconnected=off
  wires:
  Sum/1 -> Gain/1
  "Integrator, Second-Order"/1 -> Theta1/1
  d1/1 -> Sum1/2
  Gain1/1 -> Sum/2
  Va1/1 -> Sum/1  "Va1"
  Gain/1 -> Sum1/1
  Sum1/1 -> Gain2/1
  Gain2/1 -> "Integrator, Second-Order"/1  "ddTheta1"
  "Integrator, Second-Order"/2 -> Gain1/1, dTheta1/1

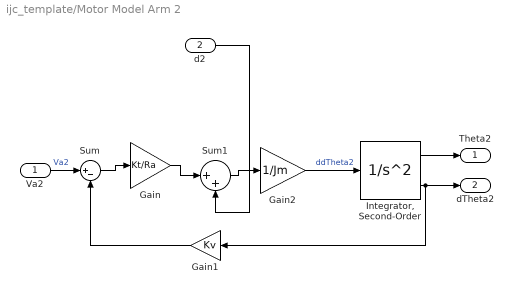
== system ijc_template/Motor Model Arm 2 ==
  Va2 : Inport
  d2 : Inport  Port=2
  Gain : Gain  Gain=Kt/Ra
  Gain1 : Gain  Gain=Kv
  Gain2 : Gain  Gain=1/Jm
  "Integrator, Second-Order" : SecondOrderIntegrator
  Sum : Sum  Inputs=|+-
  Sum1 : Sum  Inputs=|++
  Theta2 : Outport  VectorParamsAs1DForOutWhenUnconnected=off
  dTheta2 : Outport  Port=2  VectorParamsAs1DForOutWhenUnconnected=off
  wires:
  Sum/1 -> Gain/1
  "Integrator, Second-Order"/1 -> Theta2/1
  d2/1 -> Sum1/2
  "Integrator, Second-Order"/2 -> Gain1/1, dTheta2/1
  Gain1/1 -> Sum/2
  Va2/1 -> Sum/1  "Va2"
  Gain/1 -> Sum1/1
  Sum1/1 -> Gain2/1
  Gain2/1 -> "Integrator, Second-Order"/1  "ddTheta2"

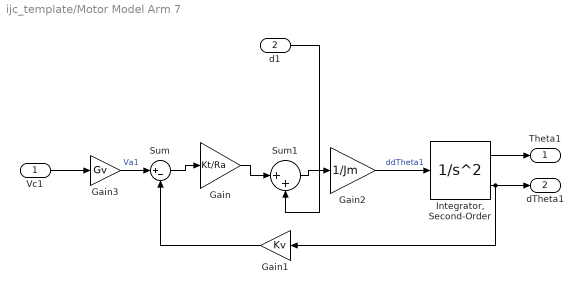
== system ijc_template/Motor Model Arm 7 ==
  Vc1 : Inport
  d1 : Inport  Port=2
  Gain : Gain  Gain=Kt/Ra
  Gain1 : Gain  Gain=Kv
  Gain2 : Gain  Gain=1/Jm
  Gain3 : Gain  Gain=Gv
  "Integrator, Second-Order" : SecondOrderIntegrator
  Sum : Sum  Inputs=|+-
  Sum1 : Sum  Inputs=|++
  Theta1 : Outport  VectorParamsAs1DForOutWhenUnconnected=off
  dTheta1 : Outport  Port=2  VectorParamsAs1DForOutWhenUnconnected=off
  wires:
  Sum/1 -> Gain/1
  "Integrator, Second-Order"/1 -> Theta1/1
  d1/1 -> Sum1/2
  Gain1/1 -> Sum/2
  Gain3/1 -> Sum/1  "Va1"
  Gain/1 -> Sum1/1
  Sum1/1 -> Gain2/1
  Gain2/1 -> "Integrator, Second-Order"/1  "ddTheta1"
  "Integrator, Second-Order"/2 -> Gain1/1, dTheta1/1
  Vc1/1 -> Gain3/1

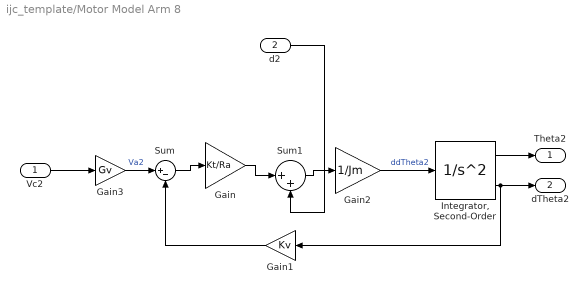
== system ijc_template/Motor Model Arm 8 ==
  Vc2 : Inport
  d2 : Inport  Port=2
  Gain : Gain  Gain=Kt/Ra
  Gain1 : Gain  Gain=Kv
  Gain2 : Gain  Gain=1/Jm
  Gain3 : Gain  Gain=Gv
  "Integrator, Second-Order" : SecondOrderIntegrator
  Sum : Sum  Inputs=|+-
  Sum1 : Sum  Inputs=|++
  Theta2 : Outport  VectorParamsAs1DForOutWhenUnconnected=off
  dTheta2 : Outport  Port=2  VectorParamsAs1DForOutWhenUnconnected=off
  wires:
  Sum/1 -> Gain/1
  "Integrator, Second-Order"/1 -> Theta2/1
  d2/1 -> Sum1/2
  "Integrator, Second-Order"/2 -> Gain1/1, dTheta2/1
  Gain1/1 -> Sum/2
  Gain3/1 -> Sum/1  "Va2"
  Gain/1 -> Sum1/1
  Sum1/1 -> Gain2/1
  Gain2/1 -> "Integrator, Second-Order"/1  "ddTheta2"
  Vc2/1 -> Gain3/1

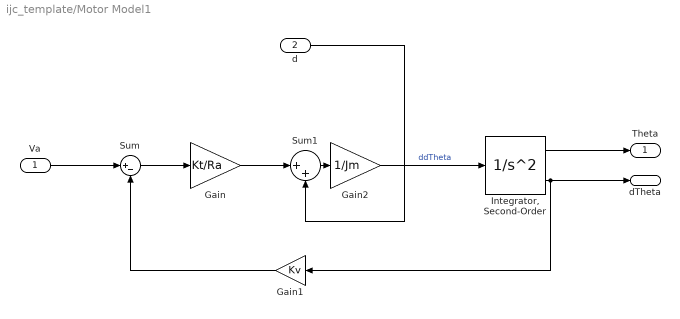
== system ijc_template/Motor Model1 ==
  Va : Inport
  d : Inport  Port=2
  Gain : Gain  Gain=Kt/Ra
  Gain1 : Gain  Gain=Kv
  Gain2 : Gain  Gain=1/Jm
  "Integrator, Second-Order" : SecondOrderIntegrator
  Sum : Sum  Inputs=|+-
  Sum1 : Sum  Inputs=|++
  Theta : Outport  VectorParamsAs1DForOutWhenUnconnected=off
  dTheta : Outport  Port=2  VectorParamsAs1DForOutWhenUnconnected=off
  wires:
  Sum/1 -> Gain/1
  "Integrator, Second-Order"/1 -> Theta/1
  d/1 -> Sum1/2
  Gain1/1 -> Sum/2
  Va/1 -> Sum/1
  Gain/1 -> Sum1/1
  Sum1/1 -> Gain2/1
  Gain2/1 -> "Integrator, Second-Order"/1  "ddTheta"
  "Integrator, Second-Order"/2 -> Gain1/1, dTheta/1

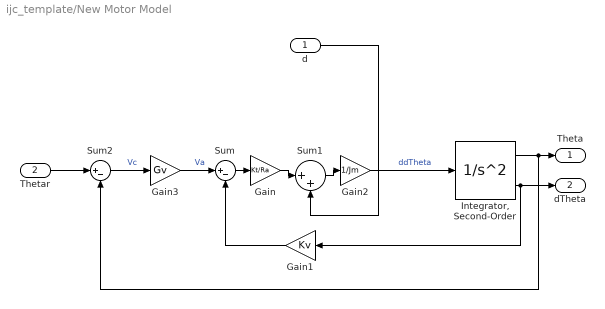
== system ijc_template/New Motor Model ==
  d : Inport
  Thetar : Inport  Port=2
  Gain : Gain  Gain=Kt/Ra
  Gain1 : Gain  Gain=Kv
  Gain2 : Gain  Gain=1/Jm
  Gain3 : Gain  Gain=Gv
  "Integrator, Second-Order" : SecondOrderIntegrator
  Sum : Sum  Inputs=|+-
  Sum1 : Sum  Inputs=|++
  Sum2 : Sum  Inputs=|+-
  Theta : Outport  VectorParamsAs1DForOutWhenUnconnected=off
  dTheta : Outport  Port=2  VectorParamsAs1DForOutWhenUnconnected=off
  wires:
  Sum/1 -> Gain/1
  "Integrator, Second-Order"/1 -> Sum2/2, Theta/1
  d/1 -> Sum1/2
  "Integrator, Second-Order"/2 -> Gain1/1, dTheta/1
  Gain1/1 -> Sum/2
  Gain3/1 -> Sum/1  "Va"
  Gain/1 -> Sum1/1
  Sum1/1 -> Gain2/1
  Gain2/1 -> "Integrator, Second-Order"/1  "ddTheta"
  Thetar/1 -> Sum2/1
  Sum2/1 -> Gain3/1  "Vc"

== matlab function ijc_template/G_matrix1 ==
  data: G output; q1 input; q2 input; g parameter; l1 parameter; lc1 parameter; lc2 parameter; m1 parameter; m2 parameter
function G = G_matrix(q1,q2, g, l1, lc1, lc2, m1, m2)
%#codegen

%    This function was generated by the Symbolic Math Toolbox version 8.3.
%    05-Nov-2019 15:18:30

t2 = cos(q1);
t3 = q1+q2;
t4 = cos(t3);
G = [g.*m2.*(l1.*t2+lc2.*t4)+g.*lc1.*m1.*t2;g.*lc2.*m2.*t4];

== matlab function ijc_template/G_matrix2 ==
  data: G output; q1 input; q2 input; g parameter; l1 parameter; lc1 parameter; lc2 parameter; m1 parameter; m2 parameter
function G = G_matrix(q1,q2, g, l1, lc1, lc2, m1, m2)
%#codegen

%    This function was generated by the Symbolic Math Toolbox version 8.3.
%    05-Nov-2019 15:18:30

t2 = cos(q1);
t3 = q1+q2;
t4 = cos(t3);
G = [g.*m2.*(l1.*t2+lc2.*t4)+g.*lc1.*m1.*t2;g.*lc2.*m2.*t4];

== matlab function ijc_template/Link Motor1/G_matrix ==
  data: G output; q1 input; q2 input; g parameter; l1 parameter; lc1 parameter; lc2 parameter; m1 parameter; m2 parameter
function G = G_matrix(q1,q2, g, l1, lc1, lc2, m1, m2)
%#codegen

%    This function was generated by the Symbolic Math Toolbox version 8.3.
%    05-Nov-2019 15:18:30

t2 = cos(q1);
t3 = q1+q2;
t4 = cos(t3);
G = [g.*m2.*(l1.*t2+lc2.*t4)+g.*lc1.*m1.*t2;g.*lc2.*m2.*t4];

== matlab function ijc_template/Link Motor/G_matrix ==
  data: G output; q1 input; q2 input; g parameter; l1 parameter; lc1 parameter; lc2 parameter; m1 parameter; m2 parameter
function G = G_matrix(q1,q2, g, l1, lc1, lc2, m1, m2)
%#codegen

%    This function was generated by the Symbolic Math Toolbox version 8.3.
%    05-Nov-2019 15:18:30

t2 = cos(q1);
t3 = q1+q2;
t4 = cos(t3);
G = [g.*m2.*(l1.*t2+lc2.*t4)+g.*lc1.*m1.*t2;g.*lc2.*m2.*t4];
